simulink model "hemZ_machine_model_modulation_changed_NO_angle_3Level"  (R2024a)
settings: Solver=VariableStepAuto  StartTime=0.0  StopTime=0.2  FixedStep=1e-7  MaxStep=1e-7  RelTol=1e-3
undefined symbols (not defined in the file or in its folder): fluxMaps, invFluxMaps, Kiid, Kiiq, Kpid, Kpiq, Ld_simp, Lq_simp, n_m, OPmaps, p, Rs, switchingStrategy, T, Ts, udc
libraries: spsTriangleGeneratorLib x15, spsFirstOrderFilterLib x2, spsSVPWMGenerator2LevelLib x1
settings Model: Creator=lbocker  LastModifiedBy=lbocker
settings DebuggingCC: SignalInfNanChecking=warning
settings RTWCC: GPUComputeCapability=3.5

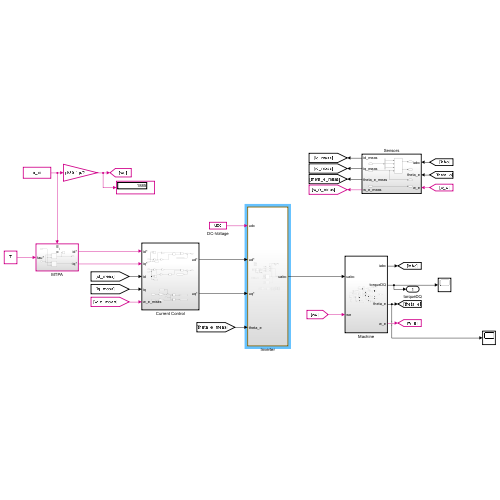
[thumbnail: Simulink's stored preview of the top-level diagram]
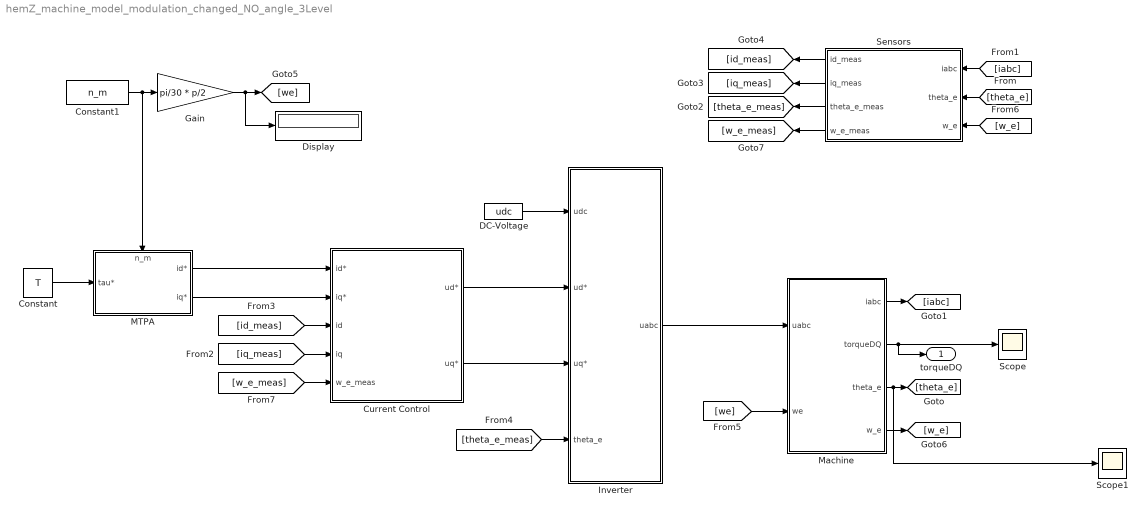
== system hemZ_machine_model_modulation_changed_NO_angle_3Level ==
  Constant : Constant  Value=T
  Constant1 : Constant  Value=n_m
  Current Control : Subsystem
  DC-Voltage : Constant  Value=udc
  Display : Display
  Gain : Gain  Gain=pi/30 * p/2
  Inverter : Subsystem
  MTPA : Subsystem
      settings: PortSchema="{\"entries\":[{\"content\":{\"sides\":[{\"content\":{\"connectorIds\":[\"In1\"]},\"type\":\"ConnectorPlacement.EquallySpacedRectSide\",\"uuid\":\"10ab731b-3e6d-43a6-a9a5-b7fbc10206be\"},{\"content\":{\"connectorIds\":[\"Out1\",\"Out2\"],\"side\":\"RIGHT\"},\"type\":\"ConnectorPlacement.EquallySpacedRectSide\",\"uuid\":\"a5a9f411-ee76-4677-8acf-be72a2146ad7\"},{\"content\":{\"connectorIds\":[\"In2\"],\"side\":\"TOP\"},\"type\":\"ConnectorPlacement.EquallySpacedRectSide\",\"uuid\":\"4655eeb1-fbf4-410e-b241-91e2c0b3f1e6\"}]},\"type\":\"ConnectorPlacement.EquallySpacedConnector\",\"uuid\":\"156083f5-90bf-4402-853e-1f267376ca38\"}],\"packageUris\":[\"http://schema.mathworks.com/mf0/Connector/R2020b\"],\"version\":\"1.0\"}"
  Machine : Subsystem
  Scope : Scope
  Scope1 : Scope
  Sensors : Subsystem
  torqueDQ : Outport
  wires:
  [we] -> Machine/2(we)
  Machine/2(torqueDQ) -> Scope/1, torqueDQ/1
  Inverter/1(uabc) -> Machine/1(uabc)
  Machine/1(iabc) -> [iabc]
  Machine/3(theta_e) -> Scope1/1, [theta_e]
  [theta_e] -> Sensors/2(theta_e)
  [iabc] -> Sensors/1(iabc)
  Sensors/3(theta_e_meas) -> [theta_e_meas]
  Sensors/2(iq_meas) -> [iq_meas]
  Sensors/1(id_meas) -> [id_meas]
  [iq_meas] -> Current Control/4(iq)
  [id_meas] -> Current Control/3(id)
  [theta_e_meas] -> Inverter/4(theta_e)
  DC-Voltage/1 -> Inverter/1(udc)
  Constant/1 -> MTPA/1(tau*)
  Constant1/1 -> MTPA/2(n_m), Gain/1
  Gain/1 -> Display/1, [we]
  Machine/4(w_e) -> [w_e]
  [w_e] -> Sensors/3(w_e)
  Sensors/4(w_e_meas) -> [w_e_meas]
  [w_e_meas] -> Current Control/5(w_e_meas)
  MTPA/1(id*) -> Current Control/1(id*)
  MTPA/2(iq*) -> Current Control/2(iq*)
  Current Control/1(ud*) -> Inverter/2(ud*)
  Current Control/2(uq*) -> Inverter/3(uq*)

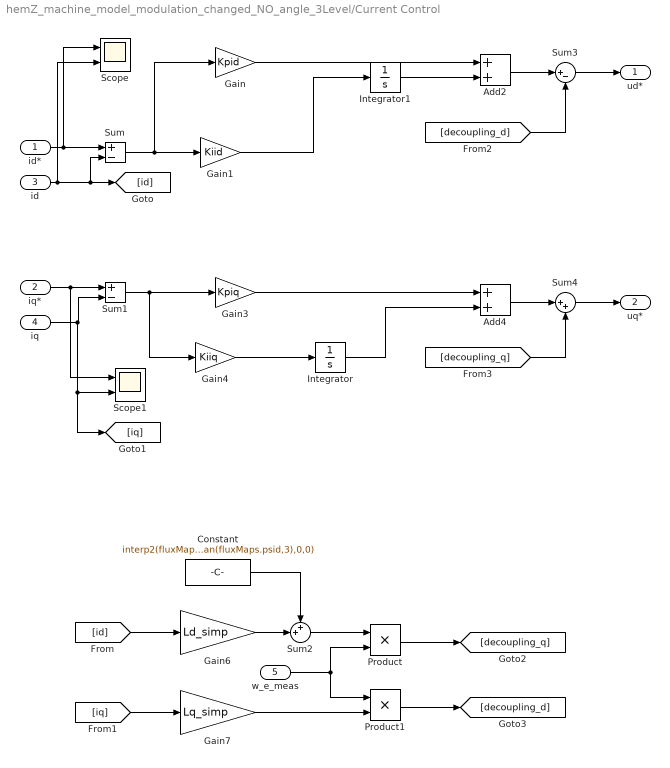
== system hemZ_machine_model_modulation_changed_NO_angle_3Level/Current Control ==
  id* : Inport
  iq* : Inport  Port=2
  id : Inport  Port=3
  iq : Inport  Port=4
  w_e_meas : Inport  Port=5
  Add2 : Sum
  Add4 : Sum
  Constant : Constant  Value=interp2(fluxMaps.id,fluxMaps.iq,mean(fluxMaps.psid,3),0,0)
  Gain : Gain  Gain=Kpid
  Gain1 : Gain  Gain=Kiid
  Gain3 : Gain  Gain=Kpiq
  Gain4 : Gain  Gain=Kiiq
  Gain6 : Gain  Gain=Ld_simp
  Gain7 : Gain  Gain=Lq_simp
  Integrator : Integrator
  Integrator1 : Integrator
  Product : Product
  Product1 : Product
  Scope : Scope  NumInputPorts=2
  Scope1 : Scope  NumInputPorts=2
  Sum : Sum  Inputs=+-
  Sum1 : Sum  Inputs=+-
  Sum2 : Sum  Inputs=++|
  Sum3 : Sum  Inputs=|+-
  Sum4 : Sum  Inputs=|++
  ud* : Outport
  uq* : Outport  Port=2
  wires:
  id*/1 -> Scope/1, Sum/1
  id/1 -> [id], Sum/2, Scope/2
  iq*/1 -> Scope1/1, Sum1/1
  iq/1 -> [iq], Scope1/2, Sum1/2
  Sum/1 -> Gain/1, Gain1/1
  Gain/1 -> Add2/1
  Gain1/1 -> Integrator1/1
  Add2/1 -> Sum3/1
  Gain3/1 -> Add4/1
  Sum1/1 -> Gain3/1, Gain4/1
  Add4/1 -> Sum4/1
  [id] -> Gain6/1
  [iq] -> Gain7/1
  Gain6/1 -> Sum2/2
  Constant/1 -> Sum2/1
  Sum2/1 -> Product/1
  w_e_meas/1 -> Product/2, Product1/1
  Gain7/1 -> Product1/2
  Product/1 -> [decoupling_q]
  Product1/1 -> [decoupling_d]
  Sum3/1 -> ud*/1
  [decoupling_d] -> Sum3/2
  Sum4/1 -> uq*/1
  [decoupling_q] -> Sum4/2
  Gain4/1 -> Integrator/1
  Integrator/1 -> Add4/2
  Integrator1/1 -> Add2/2

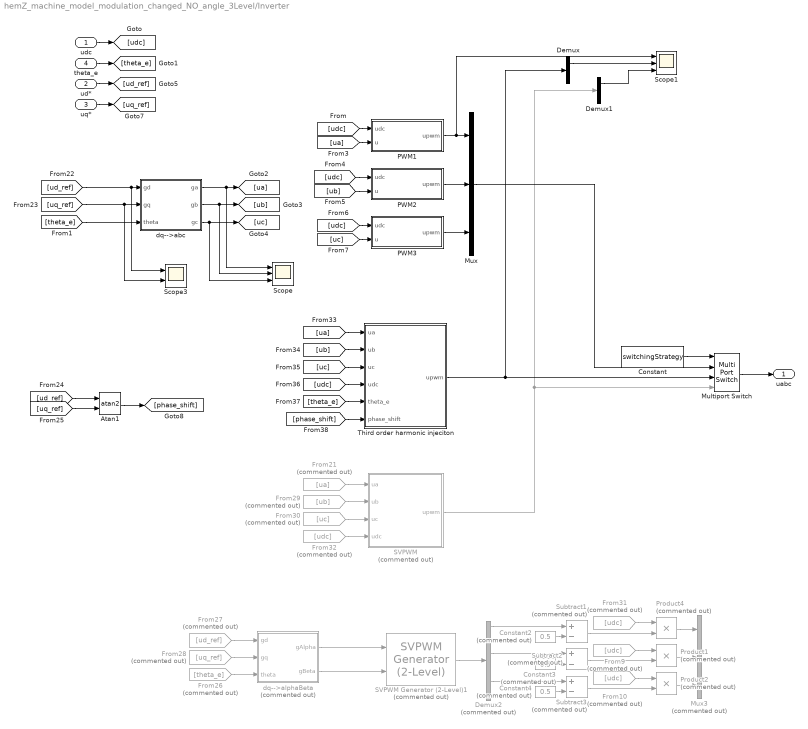
== system hemZ_machine_model_modulation_changed_NO_angle_3Level/Inverter ==
  udc : Inport
  ud* : Inport  Port=2
  uq* : Inport  Port=3
  theta_e : Inport  Port=4
  Atan1 : Trigonometry  Operator=atan2
  Constant : Constant  Value=switchingStrategy
  Constant2 : Constant  Commented=on  Value=0.5
  Constant3 : Constant  Commented=on  Value=0.5
  Constant4 : Constant  Commented=on  Value=0.5
  Demux : Demux  Outputs=3
  Demux1 : Demux  Outputs=3
  Demux2 : Demux  Commented=on  Outputs=6
  From{9..10,31..32} (4 alike) : From  Commented=on  GotoTag=udc
  From21 : From  Commented=on  GotoTag=ua
  From26 : From  Commented=on  GotoTag=theta_e
  From27 : From  Commented=on  GotoTag=ud_ref
  From28 : From  Commented=on  GotoTag=uq_ref
  From29 : From  Commented=on  GotoTag=ub
  From30 : From  Commented=on  GotoTag=uc
  Multiport Switch : MultiPortSwitch  SaturateOnIntegerOverflow=off  InputSameDT=off
  Mux : Mux  Inputs=3
  Mux3 : Mux  Commented=on  Inputs=3
  PWM1 : Subsystem
  PWM2 : Subsystem
  PWM3 : Subsystem
  Product1 : Product  Commented=on
  Product2 : Product  Commented=on
  Product4 : Product  Commented=on
  SVPWM : Subsystem  Commented=on
  SVPWM Generator (2-Level)1 : spsSVPWMGenerator2LevelLib/SVPWM Generator (2-Level)  Commented=on  InputType=alpha-beta components  SwitchingPattern=Pattern #1  Fc=1/Ts  ParUref=[0.8 -30 50]  Ts=0
  Scope : Scope  NumInputPorts=3
  Scope1 : Scope  NumInputPorts=3
  Scope3 : Scope  NumInputPorts=2
  Subtract1 : Sum  Commented=on  Inputs=+-
  Subtract2 : Sum  Commented=on  Inputs=+-
  Subtract3 : Sum  Commented=on  Inputs=+-
  Third order harmonic injeciton : Subsystem
  dq-->abc : MATLAB Function  TreatAsAtomicUnit=on
  dq-->alphaBeta : MATLAB Function  Commented=on  TreatAsAtomicUnit=on
  uabc : Outport
  wires:
  udc/1 -> [udc]
  [udc] -> PWM1/1(udc)
  [ud_ref] -> Scope3/1, dq-->abc/1(gd)
  [uq_ref] -> Scope3/2, dq-->abc/2(gq)
  theta_e/1 -> [theta_e]
  [theta_e] -> dq-->abc/3(theta)
  dq-->abc/1(ga) -> Scope/1, [ua]
  dq-->abc/2(gb) -> Scope/2, [ub]
  dq-->abc/3(gc) -> Scope/3, [uc]
  [ua] -> PWM1/2(u)
  [ub] -> PWM2/2(u)
  [udc] -> PWM2/1(udc)
  [udc] -> PWM3/1(udc)
  [uc] -> PWM3/2(u)
  PWM1/1(upwm) -> Scope1/1, Mux/1
  PWM3/1(upwm) -> Mux/3
  PWM2/1(upwm) -> Mux/2
  ud*/1 -> [ud_ref]
  uq*/1 -> [uq_ref]
  [ud_ref] -> Atan1/1
  [uq_ref] -> Atan1/2
  Atan1/1 -> [phase_shift]
  From26/1 -> dq-->alphaBeta/3(theta)
  From27/1 -> dq-->alphaBeta/1(gd)
  From28/1 -> dq-->alphaBeta/2(gq)
  dq-->alphaBeta/1(gAlpha) -> SVPWM Generator (2-Level)1/1
  dq-->alphaBeta/2(gBeta) -> SVPWM Generator (2-Level)1/2
  SVPWM Generator (2-Level)1/1 -> Demux2/1
  Demux2/1 -> Subtract1/1
  Constant2/1 -> Subtract1/2
  Constant3/1 -> Subtract2/2
  Demux2/3 -> Subtract2/1
  Constant4/1 -> Subtract3/2
  Demux2/5 -> Subtract3/1
  From31/1 -> Product4/1
  Subtract1/1 -> Product4/2
  From9/1 -> Product1/1
  Subtract2/1 -> Product1/2
  From10/1 -> Product2/1
  Subtract3/1 -> Product2/2
  Product4/1 -> Mux3/1
  Product1/1 -> Mux3/2
  Product2/1 -> Mux3/3
  Constant/1 -> Multiport Switch/1
  Multiport Switch/1 -> uabc/1
  From21/1 -> SVPWM/1(ua)
  From29/1 -> SVPWM/2(ub)
  From30/1 -> SVPWM/3(uc)
  From32/1 -> SVPWM/4(udc)
  [udc] -> Third order harmonic injeciton/4(udc)
  [uc] -> Third order harmonic injeciton/3(uc)
  [ub] -> Third order harmonic injeciton/2(ub)
  [ua] -> Third order harmonic injeciton/1(ua)
  [theta_e] -> Third order harmonic injeciton/5(theta_e)
  [phase_shift] -> Third order harmonic injeciton/6(phase_shift)
  SVPWM/1(upwm) -> Demux1/1, Multiport Switch/4
  Third order harmonic injeciton/1(upwm) -> Demux/1, Multiport Switch/3
  Demux/1 -> Scope1/2
  Demux1/1 -> Scope1/3
  Mux/1 -> Multiport Switch/2

== system hemZ_machine_model_modulation_changed_NO_angle_3Level/MTPA ==
  tau* : Inport
  n_m : Inport  Port=2
  2-D Lookup Table : Lookup_n-D  BreakpointsForDimension1=OPmaps.tau  BreakpointsForDimension2=OPmaps.n_m  Table=OPmaps.id  InternalRulePriority=Speed  RndMeth=Simplest
      settings: InputPortMap=u0,u1
  2-D Lookup Table1 : Lookup_n-D  BreakpointsForDimension1=OPmaps.tau  BreakpointsForDimension2=OPmaps.n_m  Table=OPmaps.iq  InternalRulePriority=Speed  RndMeth=Simplest
      settings: InputPortMap=u0,u1
  Scope : Scope
  id* : Outport
  iq* : Outport  Port=2
  wires:
  tau*/1 -> 2-D Lookup Table1/1, 2-D Lookup Table/1
  2-D Lookup Table/1 -> Scope/1, id*/1
  2-D Lookup Table1/1 -> iq*/1
  n_m/1 -> 2-D Lookup Table1/2, 2-D Lookup Table/2

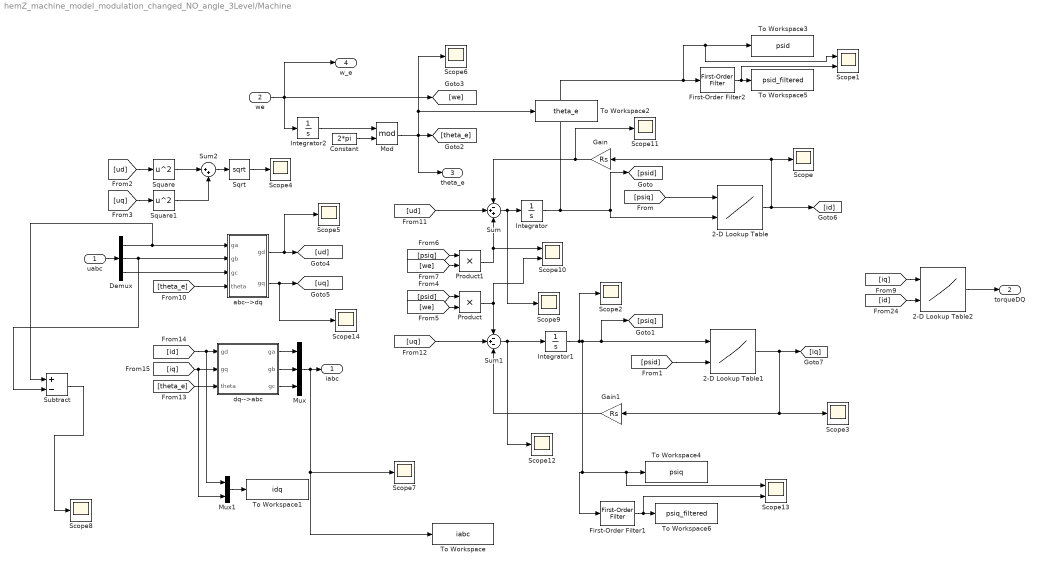
== system hemZ_machine_model_modulation_changed_NO_angle_3Level/Machine ==
  uabc : Inport
  we : Inport  Port=2
  2-D Lookup Table : Lookup_n-D  BreakpointsForDimension1=invFluxMaps.psiq  BreakpointsForDimension2=invFluxMaps.psid  Table=mean(invFluxMaps.id,3)  InternalRulePriority=Speed  RndMeth=Simplest
      settings: InputPortMap=u0,u1
  2-D Lookup Table1 : Lookup_n-D  BreakpointsForDimension1=invFluxMaps.psiq  BreakpointsForDimension2=invFluxMaps.psid  Table=mean(invFluxMaps.iq,3)  InternalRulePriority=Speed  RndMeth=Simplest
      settings: InputPortMap=u0,u1
  2-D Lookup Table2 : Lookup_n-D  BreakpointsForDimension1=fluxMaps.iq  BreakpointsForDimension2=fluxMaps.id  Table=mean(fluxMaps.tau,3)  InternalRulePriority=Speed  RndMeth=Simplest
      settings: InputPortMap=u0,u1
  Constant : Constant  Value=2*pi
  Demux : Demux  Outputs=3
  First-Order Filter1 : spsFirstOrderFilterLib/First-Order Filter  FilterType=Lowpass  Tc=1e-5  Ts=0  Initialize=on  Vac_Init=[0, 0, 60]  Vdc_Init=0  PlotResponse=off  FreqRange="[0,  200,  1]"
  First-Order Filter2 : spsFirstOrderFilterLib/First-Order Filter  FilterType=Lowpass  Tc=1e-5  Ts=0  Initialize=on  Vac_Init=[0, 0, 60]  Vdc_Init=0  PlotResponse=off  FreqRange="[0,  200,  1]"
  Gain : Gain  Gain=Rs
  Gain1 : Gain  Gain=Rs
  Integrator : Integrator  InitialCondition=interp2(fluxMaps.id,fluxMaps.iq,mean(fluxMaps.psid,3),0,0)
  Integrator1 : Integrator  InitialCondition=interp2(fluxMaps.id,fluxMaps.iq,mean(fluxMaps.psiq,3),0,0)
  Integrator2 : Integrator
  Mod : Math  Operator=mod
  Mux : Mux  Inputs=3
  Mux1 : Mux  Inputs=2
  Product : Product
  Product1 : Product
  Scope{,2..9,11..12,14} (12 alike) : Scope
  Scope1 : Scope  NumInputPorts=2
  Scope10 : Scope  NumInputPorts=2
  Scope13 : Scope  NumInputPorts=2
  Sqrt : Sqrt
  Square : Math  Operator=square
  Square1 : Math  Operator=square
  Subtract : Sum  Inputs=+-
  Sum : Sum  Inputs=-++
  Sum1 : Sum  Inputs=-+-
  Sum2 : Sum  Inputs=|++
  To Workspace : ToWorkspace  VariableName=iabc  SaveFormat=Timeseries  SampleTime=-1
  To Workspace1 : ToWorkspace  VariableName=idq  SaveFormat=Timeseries  SampleTime=-1
  To Workspace2 : ToWorkspace  VariableName=theta_e  SaveFormat=Timeseries  SampleTime=-1
  To Workspace3 : ToWorkspace  VariableName=psid  SaveFormat=Timeseries  SampleTime=-1
  To Workspace4 : ToWorkspace  VariableName=psiq  SaveFormat=Timeseries  SampleTime=-1
  To Workspace5 : ToWorkspace  VariableName=psid_filtered  SaveFormat=Timeseries  SampleTime=-1
  To Workspace6 : ToWorkspace  VariableName=psiq_filtered  SaveFormat=Timeseries  SampleTime=-1
  abc-->dq : MATLAB Function  TreatAsAtomicUnit=on
  dq-->abc : MATLAB Function  TreatAsAtomicUnit=on
  iabc : Outport
  torqueDQ : Outport  Port=2
  theta_e : Outport  Port=3
  w_e : Outport  Port=4
  wires:
  2-D Lookup Table1/1 -> Gain1/1, Scope3/1, [iq]
  [psid] -> Product/1
  [psid] -> 2-D Lookup Table1/2
  Integrator/1 -> 2-D Lookup Table/2, [psid], First-Order Filter2/1, Scope1/1, To Workspace3/1
  2-D Lookup Table/1 -> [id], Scope/1, Gain/1
  Integrator1/1 -> First-Order Filter1/1, Scope13/1, To Workspace4/1, 2-D Lookup Table1/1, [psiq], Scope2/1
  [psiq] -> 2-D Lookup Table/1
  [we] -> Product/2
  Product/1 -> Sum1/1, Scope10/2
  [psiq] -> Product1/1
  [we] -> Product1/2
  Sum1/1 -> Scope12/1, Integrator1/1
  Gain/1 -> Scope11/1, Sum/1
  we/1 -> Integrator2/1, w_e/1, [we]
  Product1/1 -> Scope10/1, Sum/3
  Gain1/1 -> Sum1/3
  [ud] -> Sum/2
  Sum/1 -> Scope9/1, Integrator/1
  [uq] -> Sum1/2
  Demux/2 -> Subtract/2, abc-->dq/2(gb)
  Demux/3 -> abc-->dq/3(gc)
  [theta_e] -> abc-->dq/4(theta)
  Demux/1 -> Subtract/1, abc-->dq/1(ga)
  uabc/1 -> Demux/1
  abc-->dq/1(gd) -> Scope5/1, [ud]
  abc-->dq/2(gq) -> Scope14/1, [uq]
  [theta_e] -> dq-->abc/3(theta)
  [id] -> Mux1/1, dq-->abc/1(gd)
  [iq] -> Mux1/2, dq-->abc/2(gq)
  dq-->abc/1(ga) -> Mux/1
  dq-->abc/2(gb) -> Mux/2
  dq-->abc/3(gc) -> Mux/3
  Mux/1 -> To Workspace/1, Scope7/1, iabc/1
  Mod/1 -> To Workspace2/1, Scope6/1, [theta_e], theta_e/1
  Constant/1 -> Mod/2
  Integrator2/1 -> Mod/1
  Mux1/1 -> To Workspace1/1
  First-Order Filter1/1 -> Scope13/2, To Workspace6/1
  First-Order Filter2/1 -> Scope1/2, To Workspace5/1
  2-D Lookup Table2/1 -> torqueDQ/1
  [iq] -> 2-D Lookup Table2/1
  [id] -> 2-D Lookup Table2/2
  [uq] -> Square1/1
  [ud] -> Square/1
  Square/1 -> Sum2/1
  Square1/1 -> Sum2/2
  Sum2/1 -> Sqrt/1
  Sqrt/1 -> Scope4/1
  Subtract/1 -> Scope8/1

== system hemZ_machine_model_modulation_changed_NO_angle_3Level/Sensors ==
  iabc : Inport
  theta_e : Inport  Port=2
  w_e : Inport  Port=3
  Demux : Demux  Outputs=3
  abc-->dq : MATLAB Function  TreatAsAtomicUnit=on
  id_meas : Outport
  iq_meas : Outport  Port=2
  theta_e_meas : Outport  Port=3
  w_e_meas : Outport  Port=4
  wires:
  abc-->dq/1(gd) -> id_meas/1
  abc-->dq/2(gq) -> iq_meas/1
  iabc/1 -> Demux/1
  theta_e/1 -> theta_e_meas/1, abc-->dq/4(theta)
  Demux/1 -> abc-->dq/1(ga)
  Demux/2 -> abc-->dq/2(gb)
  Demux/3 -> abc-->dq/3(gc)
  w_e/1 -> w_e_meas/1

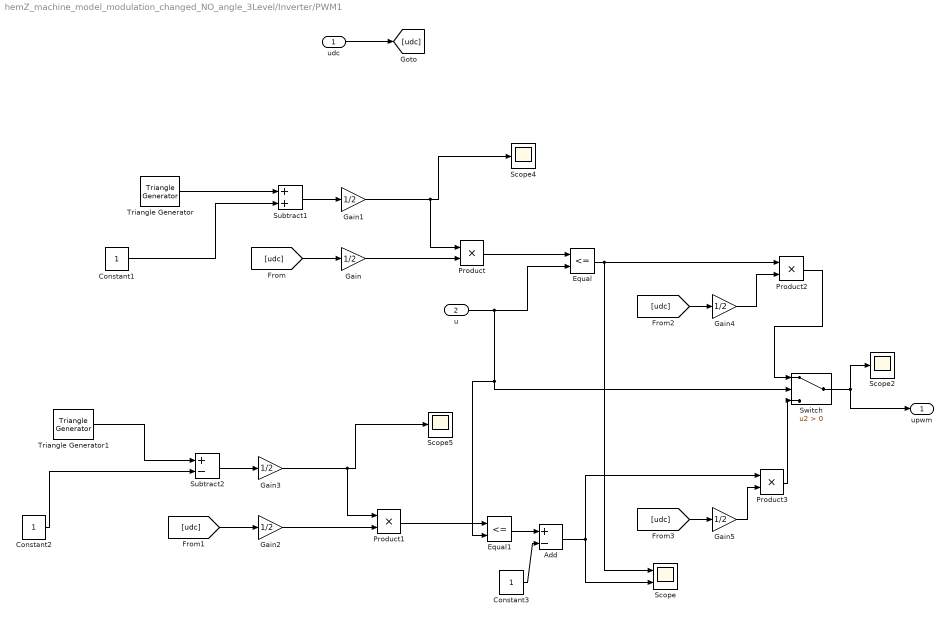
== system hemZ_machine_model_modulation_changed_NO_angle_3Level/Inverter/PWM1 ==
  udc : Inport
  u : Inport  Port=2
  Add : Sum  Inputs=+-
  Constant1 : Constant
  Constant2 : Constant
  Constant3 : Constant
  Equal : RelationalOperator  Operator=<=  OutDataTypeStr=boolean  RndMeth=Simplest  InputSameDT=off
  Equal1 : RelationalOperator  Operator=<=  OutDataTypeStr=boolean  RndMeth=Simplest  InputSameDT=off
  Gain{,1..5} (6 alike) : Gain  Gain=1/2
  Product{,1..3} (4 alike) : Product
  Scope : Scope  NumInputPorts=2
  Scope2 : Scope
  Scope4 : Scope
  Scope5 : Scope
  Subtract1 : Sum
  Subtract2 : Sum  Inputs=+-
  Switch : Switch  Criteria=u2 > Threshold  SaturateOnIntegerOverflow=off  InputSameDT=off
  Triangle Generator : spsTriangleGeneratorLib/Triangle Generator  Freq=(1/Ts)  Phase=0  Ts=0
  Triangle Generator1 : spsTriangleGeneratorLib/Triangle Generator  Freq=(1/Ts)  Phase=180  Ts=0
  upwm : Outport
  wires:
  [udc] -> Gain/1
  Product/1 -> Equal/1
  Equal/1 -> Scope/1, Product2/1
  udc/1 -> [udc]
  [udc] -> Gain4/1
  Gain/1 -> Product/2
  Triangle Generator/1 -> Subtract1/1
  Constant1/1 -> Subtract1/2
  Subtract1/1 -> Gain1/1
  Gain1/1 -> Product/1, Scope4/1
  Gain3/1 -> Product1/1, Scope5/1
  u/1 -> Switch/2, Equal1/2, Equal/2
  Triangle Generator1/1 -> Subtract2/1
  Subtract2/1 -> Gain3/1
  Gain2/1 -> Product1/2
  [udc] -> Gain2/1
  Constant2/1 -> Subtract2/2
  Product1/1 -> Equal1/1
  Equal1/1 -> Add/1
  Constant3/1 -> Add/2
  Gain4/1 -> Product2/2
  Gain5/1 -> Product3/2
  Add/1 -> Product3/1, Scope/2
  [udc] -> Gain5/1
  Product2/1 -> Switch/1
  Product3/1 -> Switch/3
  Switch/1 -> Scope2/1, upwm/1

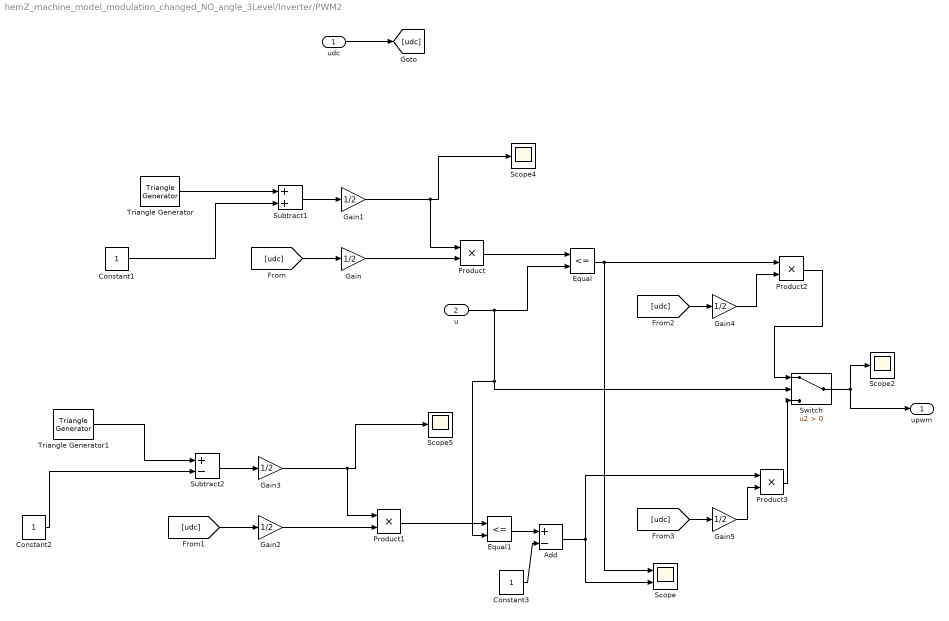
== system hemZ_machine_model_modulation_changed_NO_angle_3Level/Inverter/PWM2 ==
  udc : Inport
  u : Inport  Port=2
  Add : Sum  Inputs=+-
  Constant1 : Constant
  Constant2 : Constant
  Constant3 : Constant
  Equal : RelationalOperator  Operator=<=  OutDataTypeStr=boolean  RndMeth=Simplest  InputSameDT=off
  Equal1 : RelationalOperator  Operator=<=  OutDataTypeStr=boolean  RndMeth=Simplest  InputSameDT=off
  Gain{,1..5} (6 alike) : Gain  Gain=1/2
  Product{,1..3} (4 alike) : Product
  Scope : Scope  NumInputPorts=2
  Scope2 : Scope
  Scope4 : Scope
  Scope5 : Scope
  Subtract1 : Sum
  Subtract2 : Sum  Inputs=+-
  Switch : Switch  Criteria=u2 > Threshold  SaturateOnIntegerOverflow=off  InputSameDT=off
  Triangle Generator : spsTriangleGeneratorLib/Triangle Generator  Freq=(1/Ts)  Phase=0  Ts=0
  Triangle Generator1 : spsTriangleGeneratorLib/Triangle Generator  Freq=(1/Ts)  Phase=180  Ts=0
  upwm : Outport
  wires:
  [udc] -> Gain/1
  Product/1 -> Equal/1
  Equal/1 -> Scope/1, Product2/1
  udc/1 -> [udc]
  [udc] -> Gain4/1
  Gain/1 -> Product/2
  Triangle Generator/1 -> Subtract1/1
  Constant1/1 -> Subtract1/2
  Subtract1/1 -> Gain1/1
  Gain1/1 -> Product/1, Scope4/1
  Gain3/1 -> Product1/1, Scope5/1
  u/1 -> Switch/2, Equal1/2, Equal/2
  Triangle Generator1/1 -> Subtract2/1
  Subtract2/1 -> Gain3/1
  Gain2/1 -> Product1/2
  [udc] -> Gain2/1
  Constant2/1 -> Subtract2/2
  Product1/1 -> Equal1/1
  Equal1/1 -> Add/1
  Constant3/1 -> Add/2
  Gain4/1 -> Product2/2
  Gain5/1 -> Product3/2
  Add/1 -> Product3/1, Scope/2
  [udc] -> Gain5/1
  Product2/1 -> Switch/1
  Product3/1 -> Switch/3
  Switch/1 -> Scope2/1, upwm/1

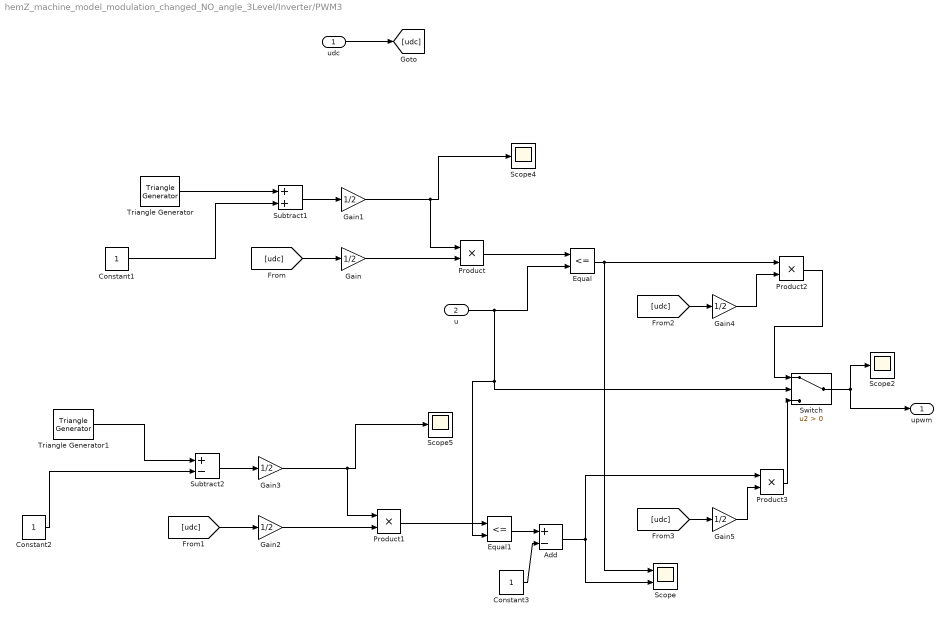
== system hemZ_machine_model_modulation_changed_NO_angle_3Level/Inverter/PWM3 ==
  udc : Inport
  u : Inport  Port=2
  Add : Sum  Inputs=+-
  Constant1 : Constant
  Constant2 : Constant
  Constant3 : Constant
  Equal : RelationalOperator  Operator=<=  OutDataTypeStr=boolean  RndMeth=Simplest  InputSameDT=off
  Equal1 : RelationalOperator  Operator=<=  OutDataTypeStr=boolean  RndMeth=Simplest  InputSameDT=off
  Gain{,1..5} (6 alike) : Gain  Gain=1/2
  Product{,1..3} (4 alike) : Product
  Scope : Scope  NumInputPorts=2
  Scope2 : Scope
  Scope4 : Scope
  Scope5 : Scope
  Subtract1 : Sum
  Subtract2 : Sum  Inputs=+-
  Switch : Switch  Criteria=u2 > Threshold  SaturateOnIntegerOverflow=off  InputSameDT=off
  Triangle Generator : spsTriangleGeneratorLib/Triangle Generator  Freq=(1/Ts)  Phase=0  Ts=0
  Triangle Generator1 : spsTriangleGeneratorLib/Triangle Generator  Freq=(1/Ts)  Phase=180  Ts=0
  upwm : Outport
  wires:
  [udc] -> Gain/1
  Product/1 -> Equal/1
  Equal/1 -> Scope/1, Product2/1
  udc/1 -> [udc]
  [udc] -> Gain4/1
  Gain/1 -> Product/2
  Triangle Generator/1 -> Subtract1/1
  Constant1/1 -> Subtract1/2
  Subtract1/1 -> Gain1/1
  Gain1/1 -> Product/1, Scope4/1
  Gain3/1 -> Product1/1, Scope5/1
  u/1 -> Switch/2, Equal1/2, Equal/2
  Triangle Generator1/1 -> Subtract2/1
  Subtract2/1 -> Gain3/1
  Gain2/1 -> Product1/2
  [udc] -> Gain2/1
  Constant2/1 -> Subtract2/2
  Product1/1 -> Equal1/1
  Equal1/1 -> Add/1
  Constant3/1 -> Add/2
  Gain4/1 -> Product2/2
  Gain5/1 -> Product3/2
  Add/1 -> Product3/1, Scope/2
  [udc] -> Gain5/1
  Product2/1 -> Switch/1
  Product3/1 -> Switch/3
  Switch/1 -> Scope2/1, upwm/1

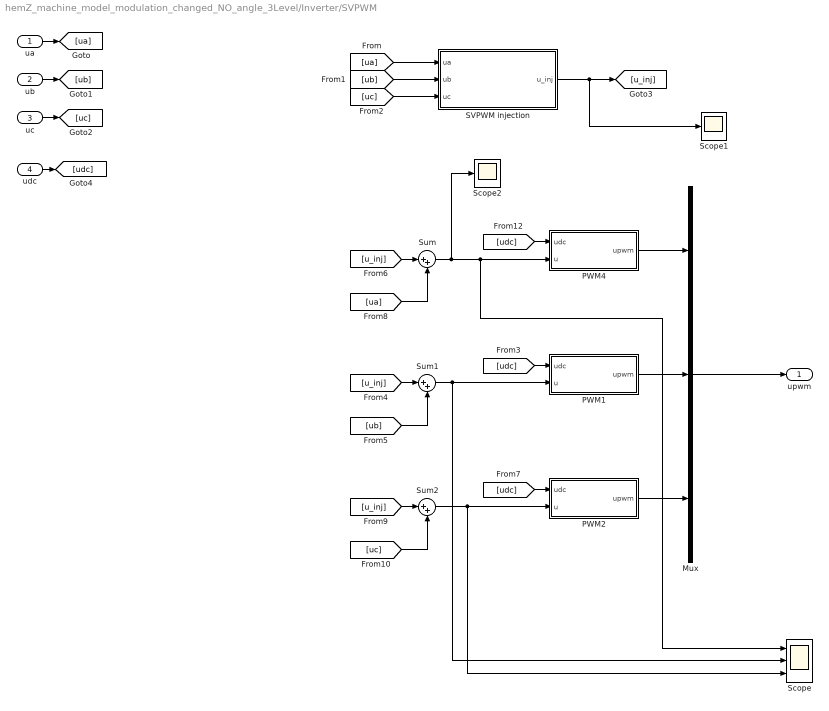
== system hemZ_machine_model_modulation_changed_NO_angle_3Level/Inverter/SVPWM ==
  ua : Inport
  ub : Inport  Port=2
  uc : Inport  Port=3
  udc : Inport  Port=4
  Mux : Mux  Inputs=3
  PWM1 : Subsystem
  PWM2 : Subsystem
  PWM4 : Subsystem
  SVPWM injection : Subsystem
  Scope : Scope  NumInputPorts=3
  Scope1 : Scope
  Scope2 : Scope
  Sum : Sum  Inputs=|++
  Sum1 : Sum  Inputs=|++
  Sum2 : Sum  Inputs=|++
  upwm : Outport
  wires:
  ua/1 -> [ua]
  ub/1 -> [ub]
  uc/1 -> [uc]
  [udc] -> PWM4/1(udc)
  [ua] -> Sum/2
  Sum/1 -> Scope2/1, Scope/1, PWM4/2(u)
  [u_inj] -> Sum/1
  udc/1 -> [udc]
  [ua] -> SVPWM injection/1(ua)
  [ub] -> SVPWM injection/2(ub)
  [uc] -> SVPWM injection/3(uc)
  PWM4/1(upwm) -> Mux/1
  [ub] -> Sum1/2
  PWM1/1(upwm) -> Mux/2
  [udc] -> PWM1/1(udc)
  [u_inj] -> Sum1/1
  Sum1/1 -> Scope/2, PWM1/2(u)
  [u_inj] -> Sum2/1
  Sum2/1 -> Scope/3, PWM2/2(u)
  [udc] -> PWM2/1(udc)
  [uc] -> Sum2/2
  PWM2/1(upwm) -> Mux/3
  Mux/1 -> upwm/1
  SVPWM injection/1(u_inj) -> Scope1/1, [u_inj]

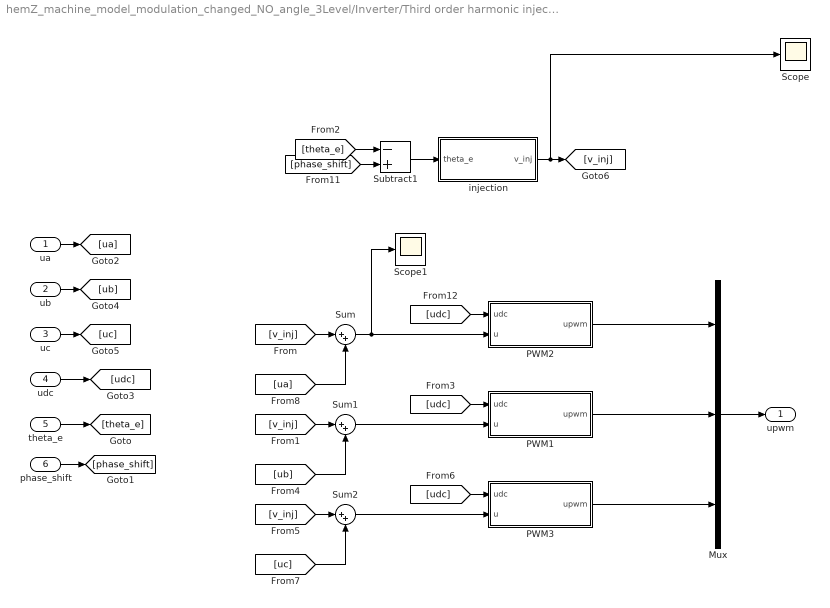
== system hemZ_machine_model_modulation_changed_NO_angle_3Level/Inverter/Third order harmonic injeciton ==
  ua : Inport
  ub : Inport  Port=2
  uc : Inport  Port=3
  udc : Inport  Port=4
  theta_e : Inport  Port=5
  phase_shift : Inport  Port=6
  Mux : Mux  Inputs=3
  PWM1 : Subsystem
  PWM2 : Subsystem
  PWM3 : Subsystem
  Scope : Scope
  Scope1 : Scope
  Subtract1 : Sum  Inputs=-+
  Sum : Sum  Inputs=|++
  Sum1 : Sum  Inputs=|++
  Sum2 : Sum  Inputs=|++
  injection : Subsystem
  upwm : Outport
  wires:
  [ua] -> Sum/2
  [theta_e] -> Subtract1/1
  [phase_shift] -> Subtract1/2
  [udc] -> PWM2/1(udc)
  Sum/1 -> PWM2/2(u), Scope1/1
  Subtract1/1 -> injection/1(theta_e)
  theta_e/1 -> [theta_e]
  phase_shift/1 -> [phase_shift]
  udc/1 -> [udc]
  ub/1 -> [ub]
  uc/1 -> [uc]
  ua/1 -> [ua]
  injection/1(v_inj) -> Scope/1, [v_inj]
  [v_inj] -> Sum/1
  [v_inj] -> Sum1/1
  Sum1/1 -> PWM1/2(u)
  [ub] -> Sum1/2
  [udc] -> PWM1/1(udc)
  Sum2/1 -> PWM3/2(u)
  [uc] -> Sum2/2
  [v_inj] -> Sum2/1
  [udc] -> PWM3/1(udc)
  PWM2/1(upwm) -> Mux/1
  PWM1/1(upwm) -> Mux/2
  PWM3/1(upwm) -> Mux/3
  Mux/1 -> upwm/1

== system hemZ_machine_model_modulation_changed_NO_angle_3Level/Inverter/SVPWM/PWM1 ==
  udc : Inport
  u : Inport  Port=2
  Constant : Constant  Value=1/2
  Equal : RelationalOperator  Operator=<=  OutDataTypeStr=boolean  RndMeth=Simplest  InputSameDT=off
  Gain : Gain  Gain=1/2
  Product : Product
  Product2 : Product
  Scope2 : Scope
  Scope3 : Scope  NumInputPorts=3
  Scope4 : Scope
  Subtract : Sum  Inputs=+-
  Triangle Generator : spsTriangleGeneratorLib/Triangle Generator  Freq=(1/Ts)  Phase=0  Ts=0
  upwm : Outport
  wires:
  Triangle Generator/1 -> Product/1, Scope4/1
  [udc] -> Gain/1
  Product/1 -> Scope3/1, Equal/1
  u/1 -> Scope3/2, Equal/2
  Subtract/1 -> Product2/1
  Product2/1 -> upwm/1, Scope2/1
  udc/1 -> [udc]
  Constant/1 -> Subtract/2
  Equal/1 -> Subtract/1, Scope3/3
  [udc] -> Product2/2
  Gain/1 -> Product/2

== system hemZ_machine_model_modulation_changed_NO_angle_3Level/Inverter/SVPWM/PWM2 ==
  udc : Inport
  u : Inport  Port=2
  Constant : Constant  Value=1/2
  Equal : RelationalOperator  Operator=<=  OutDataTypeStr=boolean  RndMeth=Simplest  InputSameDT=off
  Gain : Gain  Gain=1/2
  Product : Product
  Product2 : Product
  Scope2 : Scope
  Scope3 : Scope  NumInputPorts=3
  Scope4 : Scope
  Subtract : Sum  Inputs=+-
  Triangle Generator : spsTriangleGeneratorLib/Triangle Generator  Freq=(1/Ts)  Phase=0  Ts=0
  upwm : Outport
  wires:
  Triangle Generator/1 -> Product/1, Scope4/1
  [udc] -> Gain/1
  Product/1 -> Scope3/1, Equal/1
  u/1 -> Scope3/2, Equal/2
  Subtract/1 -> Product2/1
  Product2/1 -> upwm/1, Scope2/1
  udc/1 -> [udc]
  Constant/1 -> Subtract/2
  Equal/1 -> Subtract/1, Scope3/3
  [udc] -> Product2/2
  Gain/1 -> Product/2

== system hemZ_machine_model_modulation_changed_NO_angle_3Level/Inverter/SVPWM/PWM4 ==
  udc : Inport
  u : Inport  Port=2
  Constant : Constant  Value=1/2
  Equal : RelationalOperator  Operator=<=  OutDataTypeStr=boolean  RndMeth=Simplest  InputSameDT=off
  Gain : Gain  Gain=1/2
  Product : Product
  Product2 : Product
  Scope2 : Scope
  Scope3 : Scope  NumInputPorts=3
  Scope4 : Scope
  Subtract : Sum  Inputs=+-
  Triangle Generator : spsTriangleGeneratorLib/Triangle Generator  Freq=(1/Ts)  Phase=0  Ts=0
  upwm : Outport
  wires:
  Triangle Generator/1 -> Product/1, Scope4/1
  [udc] -> Gain/1
  Product/1 -> Scope3/1, Equal/1
  u/1 -> Scope3/2, Equal/2
  Subtract/1 -> Product2/1
  Product2/1 -> upwm/1, Scope2/1
  udc/1 -> [udc]
  Constant/1 -> Subtract/2
  Equal/1 -> Subtract/1, Scope3/3
  [udc] -> Product2/2
  Gain/1 -> Product/2

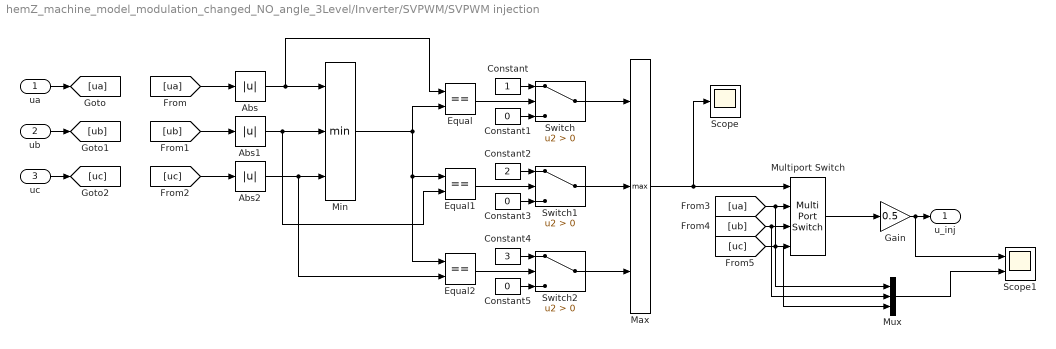
== system hemZ_machine_model_modulation_changed_NO_angle_3Level/Inverter/SVPWM/SVPWM injection ==
  ua : Inport
  ub : Inport  Port=2
  uc : Inport  Port=3
  Abs : Abs  SaturateOnIntegerOverflow=off
  Abs1 : Abs  SaturateOnIntegerOverflow=off
  Abs2 : Abs  SaturateOnIntegerOverflow=off
  Constant : Constant
  Constant1 : Constant  Value=0
  Constant2 : Constant  Value=2
  Constant3 : Constant  Value=0
  Constant4 : Constant  Value=3
  Constant5 : Constant  Value=0
  Equal : RelationalOperator  Operator===  OutDataTypeStr=boolean  RndMeth=Simplest  InputSameDT=off
  Equal1 : RelationalOperator  Operator===  OutDataTypeStr=boolean  RndMeth=Simplest  InputSameDT=off
  Equal2 : RelationalOperator  Operator===  OutDataTypeStr=boolean  RndMeth=Simplest  InputSameDT=off
  Gain : Gain  Gain=0.5
  Max : MinMax  Function=max  Inputs=3
  Min : MinMax  Inputs=3
  Multiport Switch : MultiPortSwitch  SaturateOnIntegerOverflow=off  InputSameDT=off
  Mux : Mux  Inputs=3
  Scope : Scope
  Scope1 : Scope  NumInputPorts=2
  Switch : Switch  Criteria=u2 > Threshold  SaturateOnIntegerOverflow=off  InputSameDT=off
  Switch1 : Switch  Criteria=u2 > Threshold  SaturateOnIntegerOverflow=off  InputSameDT=off
  Switch2 : Switch  Criteria=u2 > Threshold  SaturateOnIntegerOverflow=off  InputSameDT=off
  u_inj : Outport
  wires:
  Constant2/1 -> Switch1/1
  Constant5/1 -> Switch2/3
  Abs/1 -> Min/1, Equal/1
  Constant4/1 -> Switch2/1
  Min/1 -> Equal2/1, Equal1/1, Equal/2
  Constant1/1 -> Switch/3
  [uc] -> Mux/3, Multiport Switch/4
  [ub] -> Mux/2, Multiport Switch/3
  Constant/1 -> Switch/1
  Gain/1 -> Scope1/1, u_inj/1
  Switch/1 -> Max/1
  Switch1/1 -> Max/2
  Max/1 -> Scope/1, Multiport Switch/1
  Equal1/1 -> Switch1/2
  Multiport Switch/1 -> Gain/1
  Equal2/1 -> Switch2/2
  [ua] -> Mux/1, Multiport Switch/2
  Constant3/1 -> Switch1/3
  Abs1/1 -> Min/2, Equal1/2
  Switch2/1 -> Max/3
  Abs2/1 -> Min/3, Equal2/2
  Equal/1 -> Switch/2
  ub/1 -> [ub]
  uc/1 -> [uc]
  ua/1 -> [ua]
  [ua] -> Abs/1
  [ub] -> Abs1/1
  [uc] -> Abs2/1
  Mux/1 -> Scope1/2

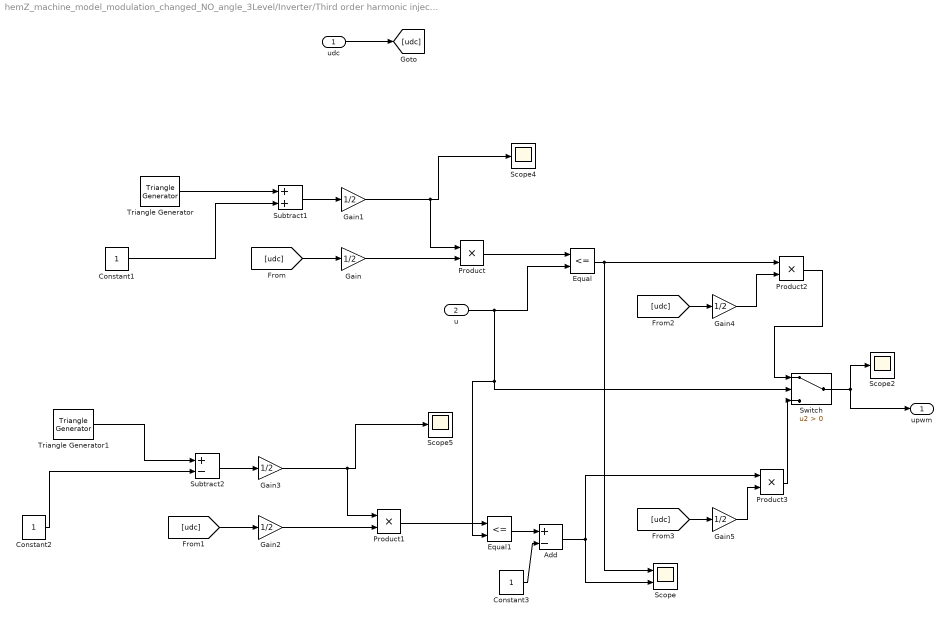
== system hemZ_machine_model_modulation_changed_NO_angle_3Level/Inverter/Third order harmonic injeciton/PWM1 ==
  udc : Inport
  u : Inport  Port=2
  Add : Sum  Inputs=+-
  Constant1 : Constant
  Constant2 : Constant
  Constant3 : Constant
  Equal : RelationalOperator  Operator=<=  OutDataTypeStr=boolean  RndMeth=Simplest  InputSameDT=off
  Equal1 : RelationalOperator  Operator=<=  OutDataTypeStr=boolean  RndMeth=Simplest  InputSameDT=off
  Gain{,1..5} (6 alike) : Gain  Gain=1/2
  Product{,1..3} (4 alike) : Product
  Scope : Scope  NumInputPorts=2
  Scope2 : Scope
  Scope4 : Scope
  Scope5 : Scope
  Subtract1 : Sum
  Subtract2 : Sum  Inputs=+-
  Switch : Switch  Criteria=u2 > Threshold  SaturateOnIntegerOverflow=off  InputSameDT=off
  Triangle Generator : spsTriangleGeneratorLib/Triangle Generator  Freq=(1/Ts)  Phase=0  Ts=0
  Triangle Generator1 : spsTriangleGeneratorLib/Triangle Generator  Freq=(1/Ts)  Phase=180  Ts=0
  upwm : Outport
  wires:
  [udc] -> Gain/1
  Product/1 -> Equal/1
  Equal/1 -> Scope/1, Product2/1
  udc/1 -> [udc]
  [udc] -> Gain4/1
  Gain/1 -> Product/2
  Triangle Generator/1 -> Subtract1/1
  Constant1/1 -> Subtract1/2
  Subtract1/1 -> Gain1/1
  Gain1/1 -> Product/1, Scope4/1
  Gain3/1 -> Product1/1, Scope5/1
  u/1 -> Switch/2, Equal1/2, Equal/2
  Triangle Generator1/1 -> Subtract2/1
  Subtract2/1 -> Gain3/1
  Gain2/1 -> Product1/2
  [udc] -> Gain2/1
  Constant2/1 -> Subtract2/2
  Product1/1 -> Equal1/1
  Equal1/1 -> Add/1
  Constant3/1 -> Add/2
  Gain4/1 -> Product2/2
  Gain5/1 -> Product3/2
  Add/1 -> Product3/1, Scope/2
  [udc] -> Gain5/1
  Product2/1 -> Switch/1
  Product3/1 -> Switch/3
  Switch/1 -> Scope2/1, upwm/1

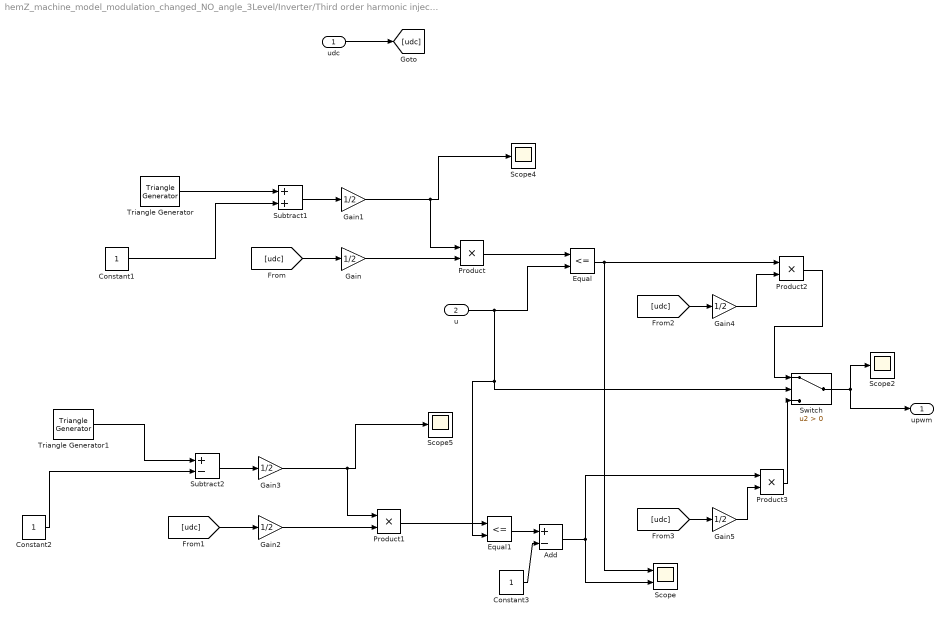
== system hemZ_machine_model_modulation_changed_NO_angle_3Level/Inverter/Third order harmonic injeciton/PWM2 ==
  udc : Inport
  u : Inport  Port=2
  Add : Sum  Inputs=+-
  Constant1 : Constant
  Constant2 : Constant
  Constant3 : Constant
  Equal : RelationalOperator  Operator=<=  OutDataTypeStr=boolean  RndMeth=Simplest  InputSameDT=off
  Equal1 : RelationalOperator  Operator=<=  OutDataTypeStr=boolean  RndMeth=Simplest  InputSameDT=off
  Gain{,1..5} (6 alike) : Gain  Gain=1/2
  Product{,1..3} (4 alike) : Product
  Scope : Scope  NumInputPorts=2
  Scope2 : Scope
  Scope4 : Scope
  Scope5 : Scope
  Subtract1 : Sum
  Subtract2 : Sum  Inputs=+-
  Switch : Switch  Criteria=u2 > Threshold  SaturateOnIntegerOverflow=off  InputSameDT=off
  Triangle Generator : spsTriangleGeneratorLib/Triangle Generator  Freq=(1/Ts)  Phase=0  Ts=0
  Triangle Generator1 : spsTriangleGeneratorLib/Triangle Generator  Freq=(1/Ts)  Phase=180  Ts=0
  upwm : Outport
  wires:
  [udc] -> Gain/1
  Product/1 -> Equal/1
  Equal/1 -> Scope/1, Product2/1
  udc/1 -> [udc]
  [udc] -> Gain4/1
  Gain/1 -> Product/2
  Triangle Generator/1 -> Subtract1/1
  Constant1/1 -> Subtract1/2
  Subtract1/1 -> Gain1/1
  Gain1/1 -> Product/1, Scope4/1
  Gain3/1 -> Product1/1, Scope5/1
  u/1 -> Switch/2, Equal1/2, Equal/2
  Triangle Generator1/1 -> Subtract2/1
  Subtract2/1 -> Gain3/1
  Gain2/1 -> Product1/2
  [udc] -> Gain2/1
  Constant2/1 -> Subtract2/2
  Product1/1 -> Equal1/1
  Equal1/1 -> Add/1
  Constant3/1 -> Add/2
  Gain4/1 -> Product2/2
  Gain5/1 -> Product3/2
  Add/1 -> Product3/1, Scope/2
  [udc] -> Gain5/1
  Product2/1 -> Switch/1
  Product3/1 -> Switch/3
  Switch/1 -> Scope2/1, upwm/1

== system hemZ_machine_model_modulation_changed_NO_angle_3Level/Inverter/Third order harmonic injeciton/PWM3 ==
  udc : Inport
  u : Inport  Port=2
  Add : Sum  Inputs=+-
  Constant1 : Constant
  Constant2 : Constant
  Constant3 : Constant
  Equal : RelationalOperator  Operator=<=  OutDataTypeStr=boolean  RndMeth=Simplest  InputSameDT=off
  Equal1 : RelationalOperator  Operator=<=  OutDataTypeStr=boolean  RndMeth=Simplest  InputSameDT=off
  Gain{,1..5} (6 alike) : Gain  Gain=1/2
  Product{,1..3} (4 alike) : Product
  Scope : Scope  NumInputPorts=2
  Scope2 : Scope
  Scope4 : Scope
  Scope5 : Scope
  Subtract1 : Sum
  Subtract2 : Sum  Inputs=+-
  Switch : Switch  Criteria=u2 > Threshold  SaturateOnIntegerOverflow=off  InputSameDT=off
  Triangle Generator : spsTriangleGeneratorLib/Triangle Generator  Freq=(1/Ts)  Phase=0  Ts=0
  Triangle Generator1 : spsTriangleGeneratorLib/Triangle Generator  Freq=(1/Ts)  Phase=180  Ts=0
  upwm : Outport
  wires:
  [udc] -> Gain/1
  Product/1 -> Equal/1
  Equal/1 -> Scope/1, Product2/1
  udc/1 -> [udc]
  [udc] -> Gain4/1
  Gain/1 -> Product/2
  Triangle Generator/1 -> Subtract1/1
  Constant1/1 -> Subtract1/2
  Subtract1/1 -> Gain1/1
  Gain1/1 -> Product/1, Scope4/1
  Gain3/1 -> Product1/1, Scope5/1
  u/1 -> Switch/2, Equal1/2, Equal/2
  Triangle Generator1/1 -> Subtract2/1
  Subtract2/1 -> Gain3/1
  Gain2/1 -> Product1/2
  [udc] -> Gain2/1
  Constant2/1 -> Subtract2/2
  Product1/1 -> Equal1/1
  Equal1/1 -> Add/1
  Constant3/1 -> Add/2
  Gain4/1 -> Product2/2
  Gain5/1 -> Product3/2
  Add/1 -> Product3/1, Scope/2
  [udc] -> Gain5/1
  Product2/1 -> Switch/1
  Product3/1 -> Switch/3
  Switch/1 -> Scope2/1, upwm/1

== system hemZ_machine_model_modulation_changed_NO_angle_3Level/Inverter/Third order harmonic injeciton/injection ==
  theta_e : Inport
  Gain : Gain  Gain=3
  Gain1 : Gain  Gain=udc/6
  Scope : Scope
  Scope2 : Scope
  Sin : Trigonometry
  v_inj : Outport
  wires:
  theta_e/1 -> Scope2/1, Gain/1
  Sin/1 -> Gain1/1
  Gain1/1 -> Scope/1, v_inj/1
  Gain/1 -> Sin/1

== matlab function hemZ_machine_model_modulation_changed_NO_angle_3Level/Inverter/dq-->abc ==
  data: gd input; ga output; gq input; theta input; gb output; gc output
function [ga,gb,gc] = fcn(gd,gq,theta)

T = [cos(theta)             -sin(theta)         ;...
     cos(theta-(2*pi/3))    -sin(theta-(2*pi/3));...
     cos(theta-(4*pi/3))    -sin(theta-(4*pi/3))];

gdq0 = [gd gq];
gabc = T*gdq0';
ga = gabc(1);
gb = gabc(2);
gc = gabc(3);
end

== matlab function hemZ_machine_model_modulation_changed_NO_angle_3Level/Machine/dq-->abc ==
  data: gd input; ga output; gq input; theta input; gb output; gc output
function [ga,gb,gc] = fcn(gd,gq,theta)

T = [cos(theta)             -sin(theta)         ;...
     cos(theta-(2*pi/3))    -sin(theta-(2*pi/3));...
     cos(theta-(4*pi/3))    -sin(theta-(4*pi/3))];

gdq0 = [gd gq];
gabc = T*gdq0';
ga = gabc(1);
gb = gabc(2);
gc = gabc(3);
end

== matlab function hemZ_machine_model_modulation_changed_NO_angle_3Level/Machine/abc-->dq ==
  data: ga input; gd output; gb input; gc input; theta input; gq output
function [gd,gq] = fcn(ga,gb,gc,theta)

T = (2/3) * [cos(theta)     cos(theta-(2*pi/3))     cos(theta-(4*pi/3));...
            -sin(theta)    -sin(theta-(2*pi/3))    -sin(theta-(4*pi/3));...
            (1/2)           (1/2)                   (1/2)];
gabc = [ga gb gc];
gdq = T*gabc';
gd = gdq(1);
gq = gdq(2);
end

== matlab function hemZ_machine_model_modulation_changed_NO_angle_3Level/Sensors/abc-->dq ==
  data: ga input; gd output; gb input; gc input; theta input; gq output
function [gd,gq] = fcn(ga,gb,gc,theta)

T = (2/3) * [cos(theta)     cos(theta-(2*pi/3))     cos(theta-(4*pi/3));...
            -sin(theta)    -sin(theta-(2*pi/3))    -sin(theta-(4*pi/3));...
            (1/2)           (1/2)                   (1/2)];
gabc = [ga gb gc];
gdq = T*gabc';
gd = gdq(1);
gq = gdq(2);
end

== matlab function hemZ_machine_model_modulation_changed_NO_angle_3Level/Inverter/dq-->alphaBeta ==
  data: gd input; gAlpha output; gq input; theta input; gBeta output
function [gAlpha,gBeta] = fcn(gd,gq,theta)

T = [cos(theta)    -sin(theta);...
     sin(theta)    cos(theta)];

gdq0 = [gd gq];
gabc = T*gdq0';
gAlpha = gabc(1);
gBeta = gabc(2);
end
